simulink model "a"  (Simulink 7.6)
settings: Solver=ode45  StartTime=0.0  StopTime=10.0  RelTol=1e-3
undefined symbols (not defined in the file): get, One, randint, sided
libraries: commdigbbndfm2 x3, dspsnks4 x3, commblkcod2 x2, commchan3 x1, commrandsrc2 x1, simulink x1, commsink2 x1, commdigbbndcpm2 x1, dspsrcs4 x1
settings Model: Creator=zhangling  LastModifiedBy=admin

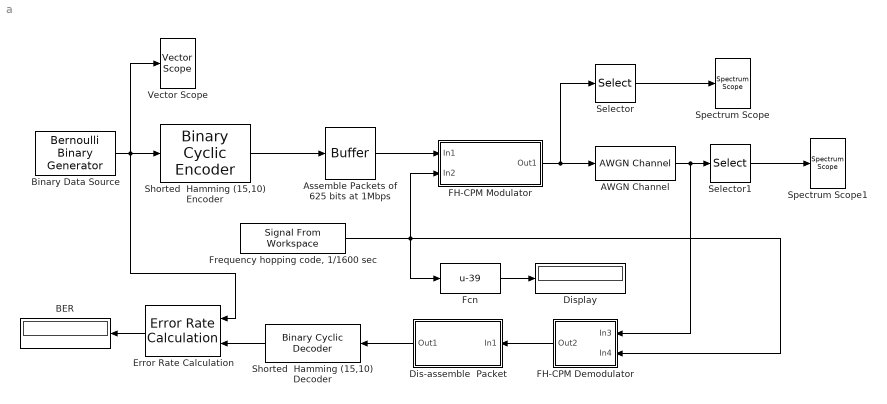
== system a ==
  AWGN Channel : commchan3/AWGN Channel  SystemSampleTime=-1  InputProcessing=Inherited (this choice will be removed - see release notes)  seed=1  noiseMode="Signal to noise ratio  (Eb/No)"  EbNodB=20  EsNodB=20  SNRdB=10  bitsPerSym=1  Ps=1  Tsym=1e-6  variance=1
  Assemble Packets of 625 bits at 1Mbps : Buffer  N=625  TreatMby1Signals=One channel
  BER : Display
  Binary Data Source : commrandsrc2/Bernoulli Binary Generator  DialogController=commDDGCreate  DialogControllerArgs=DataTag1  SystemSampleTime=-1  P=[0.5]  seed=[12345]  Ts=1.5e-6  frameBased=on  sampPerFrame=10  orient=off  outDataType=double
  Dis-assemble  Packet : Subsystem
  Display : Display
  Error Rate Calculation : commsink2/Error Rate Calculation  N=850  st_delay=0  cp_mode=Entire frame  subframe=[]  PMode=Port  WsName=ErrorVec  RsMode2=off  stop=off  numErr=100  maxBits=1e6
  FH-CPM Demodulator : Subsystem
  FH-CPM Modulator : Subsystem
  Fcn : Fcn  Expr=u-39
  "Frequency hopping code, 1/1600 sec " : dspsrcs4/Signal From Workspace  SystemSampleTime=-1  X=randint(1,100,78)  Ts=1/1600  nsamps=1  OutputAfterFinalValue=Cyclic repetition  ignoreOrWarnInputAndFrameLengths=off
  Selector : Selector  NumberOfDimensions=2  InputPortWidth=3  IndexOptions=Index vector (dialog),Index vector (dialog)  Indices=1:512,1  OutputSizes=1,1
  Selector1 : Selector  NumberOfDimensions=2  InputPortWidth=3  IndexOptions=Index vector (dialog),Index vector (dialog)  Indices=1:512,1  OutputSizes=1,1
  Shorted  Hamming (15,10) Decoder : commblkcod2/Binary Cyclic Decoder  SystemSampleTime=-1  n=7  p=4
  Shorted  Hamming (15,10) Encoder : commblkcod2/Binary Cyclic Encoder  SystemSampleTime=-1  n=15  p=[1 1 0 1 0 1]
  Spectrum Scope : dspsnks4/Spectrum Scope  DialogController=dspdialog.SpectrumScope  DialogControllerArgs=DataTag7  SystemSampleTime=-1  ScopeProperties=on  Domain=Frequency  HorizSpan=1  UseBuffer=off  BufferSize=128  Overlap=64  inpFftLenInherit=off  FFTlength=128  numAvg=2  DisplayProperties=off  AxisGrid=on  Memory=off  FrameNumber=on  AxisLegend=off  AxisZoom=off  OpenScopeAtSimStart=on  OpenScopeImmediately=off  FigPos=get(0,'defaultfigureposition')  AxisProperties=off  XUnits=Hertz  XRange=One-sided ([0...Fs/2])  XDisplay=0  InheritXIncr=on  XIncr=1.0  XLabel=Samples  XLimit=Auto  YUnits=dBW/Hertz  XMax=1  XMin=0  YLabel=Magnitude-squared, dB  LineProperties=off  wintypeSpecScope=Hann  RsSpecScope=50  betaSpecScope=5  winsampSpecScope=Periodic  XAxisParamsVer=6.9
      settings: YMin=-10  YMax=10
  Spectrum Scope1 : dspsnks4/Spectrum Scope  DialogController=dspdialog.SpectrumScope  DialogControllerArgs=DataTag8  SystemSampleTime=-1  ScopeProperties=on  Domain=Frequency  HorizSpan=1  UseBuffer=off  BufferSize=128  Overlap=64  inpFftLenInherit=off  FFTlength=128  numAvg=2  DisplayProperties=off  AxisGrid=on  Memory=off  FrameNumber=on  AxisLegend=off  AxisZoom=off  OpenScopeAtSimStart=on  OpenScopeImmediately=off  FigPos=get(0,'defaultfigureposition')  AxisProperties=off  XUnits=Hertz  XRange=One-sided ([0...Fs/2])  XDisplay=0  InheritXIncr=on  XIncr=1.0  XLabel=Samples  XLimit=Auto  YUnits=dBW/Hertz  XMax=1  XMin=0  YLabel=Magnitude-squared, dB  LineProperties=off  wintypeSpecScope=Hann  RsSpecScope=50  betaSpecScope=5  winsampSpecScope=Periodic  XAxisParamsVer=6.9
      settings: YMin=-10  YMax=10
  Vector Scope : dspsnks4/Vector Scope  DialogController=dspdialog.VectorScope  DialogControllerArgs=DataTag9  ScopeProperties=on  Domain=Time  HorizSpan=1  DisplayProperties=off  AxisGrid=on  Memory=off  FrameNumber=on  AxisLegend=off  AxisZoom=off  OpenScopeAtSimStart=on  OpenScopeImmediately=off  FigPos=get(0,'defaultfigureposition')  AxisProperties=off  XUnits=Hertz  XRange=[0...Fs/2]  InheritXIncr=on  XIncr=1  XLabel=Time  XLimit=Auto  XMin=0  XMax=1  XStart=0  YUnits=dB  YLabel=Amplitude  LineProperties=off  XAxisParamsVer=6.9
      settings: YMin=-10  YMax=10
  wires:
  Binary Data Source/1 -> Shorted  Hamming (15,10) Encoder/1, Error Rate Calculation/1, Vector Scope/1
  Shorted  Hamming (15,10) Encoder/1 -> Assemble Packets of 625 bits at 1Mbps/1
  Assemble Packets of 625 bits at 1Mbps/1 -> FH-CPM Modulator/1(In1)
  FH-CPM Modulator/1(Out1) -> AWGN Channel/1, Selector/1
  "Frequency hopping code, 1/1600 sec "/1 -> Fcn/1, FH-CPM Modulator/2(In2), FH-CPM Demodulator/2(In4)
  Selector/1 -> Spectrum Scope/1
  AWGN Channel/1 -> Selector1/1, FH-CPM Demodulator/1(In3)
  Selector1/1 -> Spectrum Scope1/1
  Fcn/1 -> Display/1
  Dis-assemble  Packet/1(Out1) -> Shorted  Hamming (15,10) Decoder/1
  Shorted  Hamming (15,10) Decoder/1 -> Error Rate Calculation/2
  Error Rate Calculation/1 -> BER/1
  FH-CPM Demodulator/1(Out2) -> Dis-assemble  Packet/1(In1)

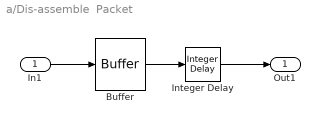
== system a/Dis-assemble  Packet ==
  In1 : Inport
  Buffer : Buffer  N=15
  Integer Delay : simulink/Discrete/Integer Delay  NumDelays=10  InputProcessing=Inherited  vinit=0.0  samptime=-1
  Out1 : Outport
  wires:
  In1/1 -> Buffer/1
  Buffer/1 -> Integer Delay/1
  Integer Delay/1 -> Out1/1

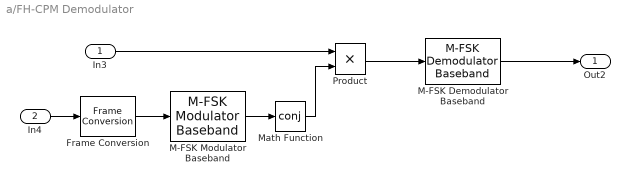
== system a/FH-CPM Demodulator ==
  In3 : Inport
  In4 : Inport  Port=2
  Frame Conversion : FrameConversion
  M-FSK Demodulator Baseband : commdigbbndfm2/M-FSK Demodulator Baseband  M=2  OutType=Bit  Dec=Binary  freqSep=10  numSamp=100  RateOptions=Inherit from input (this choice will be removed - see release notes)  outDataType=double
  M-FSK Modulator Baseband : commdigbbndfm2/M-FSK Modulator Baseband  M=79  InType=Integer  Enc=Binary  freqSep=1e6  phaseType=Continuous  numSamp=6.25e4  RateOptions=Inherit from input (this choice will be removed - see release notes)  outDataType=double
  Math Function : Math  Operator=conj  SaturateOnIntegerOverflow=on
  Product : Product  RndMeth=Zero
  Out2 : Outport
  wires:
  Product/1 -> M-FSK Demodulator Baseband/1
  Frame Conversion/1 -> M-FSK Modulator Baseband/1
  M-FSK Modulator Baseband/1 -> Math Function/1
  M-FSK Demodulator Baseband/1 -> Out2/1
  In4/1 -> Frame Conversion/1
  In3/1 -> Product/1
  Math Function/1 -> Product/2

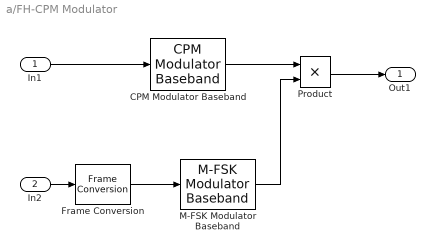
== system a/FH-CPM Modulator ==
  In1 : Inport
  In2 : Inport  Port=2
  CPM Modulator Baseband : commdigbbndcpm2/CPM Modulator Baseband  Mnum=2  inputType=Bit  mappingType=Binary  modIdx=0.3  pulseShape=Gaussian  BT=0.5  mainLobePulseLength=1  rollOff=0.2  pulseLength=1  preHistory=1  phaseOffset=0  samplesPerSymbol=8  RateOptions=Inherit from input (this choice will be removed - see release notes)  outDataType=double
  Frame Conversion : FrameConversion
  M-FSK Modulator Baseband : commdigbbndfm2/M-FSK Modulator Baseband  M=79  InType=Integer  Enc=Binary  freqSep=1e6  phaseType=Continuous  numSamp=6.25e4  RateOptions=Enforce single-rate processing  outDataType=double
  Product : Product  RndMeth=Zero
  Out1 : Outport
  wires:
  In1/1 -> CPM Modulator Baseband/1
  CPM Modulator Baseband/1 -> Product/1
  Product/1 -> Out1/1
  M-FSK Modulator Baseband/1 -> Product/2
  In2/1 -> Frame Conversion/1
  Frame Conversion/1 -> M-FSK Modulator Baseband/1
